simulink model "AM_V1"  (R2022a)
settings: Solver=VariableStepAuto  StartTime=0.0  StopTime=10.0  RelTol=1e-3
settings Model: Creator=Yogesh  LastModifiedBy=Yogesh

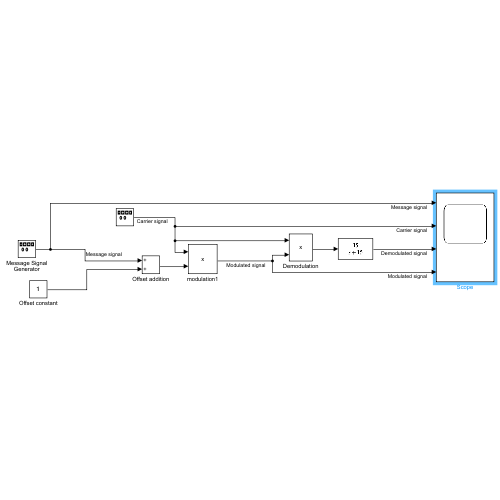
[thumbnail: Simulink's stored preview of the top-level diagram]
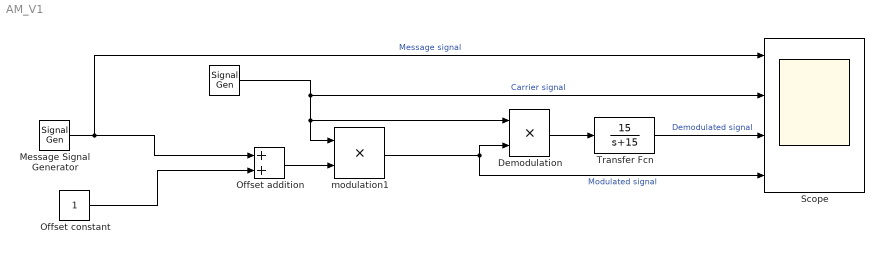
== system AM_V1 ==
  " " : SignalGenerator  Frequency=2*pi*25  Units=rad/sec
  Demodulation : Product
  Message Signal Generator : SignalGenerator  Frequency=2*pi  Units=rad/sec
  Offset addition : Sum
  Offset constant : Constant
  Scope : Scope  NumInputPorts=4
  Transfer Fcn : TransferFcn  Numerator=[15]  Denominator=[1 15]
  modulation1 : Product
  wires:
  " "/1 -> Scope/2, Demodulation/1, modulation1/1  "Carrier signal"
  Offset addition/1 -> modulation1/2
  modulation1/1 -> Demodulation/2, Scope/4  "Modulated signal"
  Message Signal Generator/1 -> Offset addition/1, Scope/1  "Message signal"
  Offset constant/1 -> Offset addition/2
  Demodulation/1 -> Transfer Fcn/1
  Transfer Fcn/1 -> Scope/3  "Demodulated signal"
